simulink model "model_wind_open_loop"  (R2020a)
settings: Solver=ode15s  StartTime=0.0  StopTime=200  MaxStep=1/60  RelTol=1e-2  AbsTol=1e-1  EnableMultiTasking=on
PreLoadFcn:
  | %load_Nordic32_data;
values from neighbouring files (symbols this model uses):
  fn = 50    [load_data_wind_open_loop.m]
  pstep = pstep_(i)    [main_wind_open_loop.m]
  time_event = 45    [load_data_wind_open_loop.m]
  wind_turbines = table(BUS,BSKV,MBASE,POPT,V_WIND,ROT_OPT, ROT_RATED)    [load_data_wind_open_loop.m]
libraries: Nordic32_Lib x2, powerlib x2
settings Model: Creator=Innocent  LastModifiedBy=joakbj
settings SolverCC: AutoScaleAbsTol=off  MaxOrder=2  ZeroCrossAlgorithm=Adaptive
settings DataIOCC: SaveFormat=Array  SaveOutput=off  SaveTime=off  ReturnWorkspaceOutputs=off
settings OptimizationCC: BlockReduction=off  BooleanDataType=off  ExpressionDepthLimit=2147483647  InitFltsAndDblsToZero=on  LifeSpan=inf
settings DebuggingCC: AlgebraicLoopMsg=none  SaveWithParameterizedLinksMsg=none  UnderspecifiedInitializationDetection=Classic  MergeDetectMultiDrivingBlocksExec=none  SignalResolutionControl=TryResolveAllWithWarning  IgnoredZcDiagnostic=none  MultiTaskDSMMsg=warning  MultiTaskCondExecSysMsg=none  FcnCallInpInsideContextMsg=warning  UnconnectedInputMsg=none  UnconnectedOutputMsg=none  UnconnectedLineMsg=none  StateNameClashWarn=warning  StrictBusMsg=ErrorOnBusTreatedAsVector  SFUnexpectedBacktrackingDiag=warning  SFNoUnconditionalDefaultTransitionDiag=warning  SFExecutionAtInitializationDiag=none  ArithmeticOperatorsInVariantConditions=warning
settings HardwareCC: ProdBitPerPointer=32  ProdBitPerSizeT=32  ProdBitPerPtrDiffT=32  ProdLargestAtomicFloat=None  ProdIntDivRoundTo=Undefined  ProdEndianess=Unspecified  ProdWordSize=32  ProdHWDeviceType=32-bit Generic
settings ModelReferenceCC: PropagateSignalLabelsOutOfModel=off
settings SFSimCC: SimUseLocalCustomCode=off  CustomCodeUndefinedFunction=UseInterfaceOnly
settings RTWCC: RTWUseLocalCustomCode=off
settings CodeAppCC: StateflowObjectComments=on
settings GRTTargetCC: TargetFcnLib=ansi_tfl_tmw.mat  TargetLangStandard=C89/C90 (ANSI)  CombineOutputUpdateFcns=off  GRTInterface=on
settings ConfigComp: CovMetricSettings=dw  CovHtmlReporting=on  CovSaveCumulativeToWorkspaceVar=on  CovSaveSingleToWorkspaceVar=on  CovExternalEMLEnable=off
settings SimscapeCC: SimscapeNormalizeSystem=off

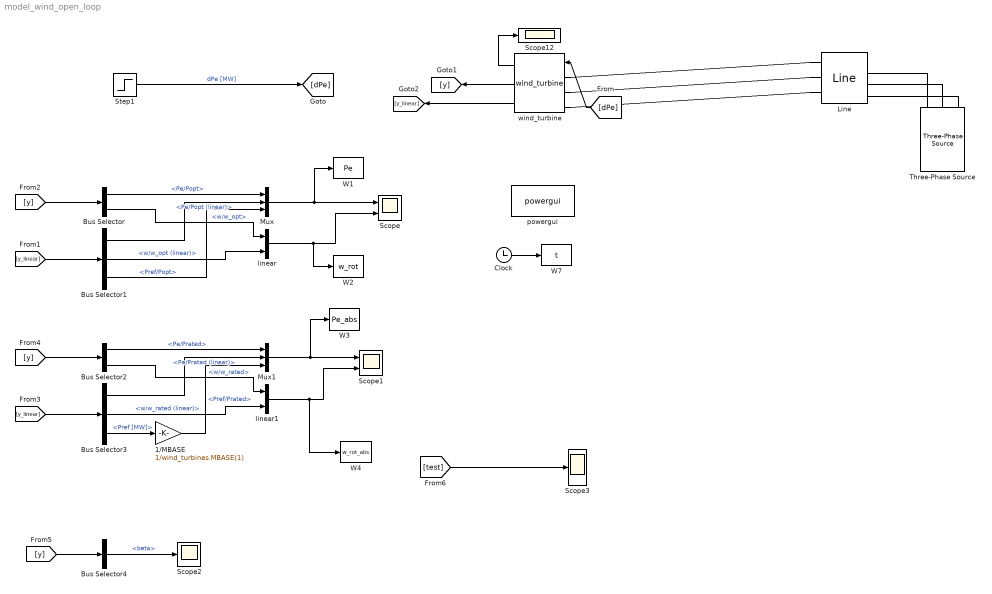
== system model_wind_open_loop ==
  1/MBASE : Gain  Gain=1/wind_turbines.MBASE(1)
  Bus Selector : BusSelector  OutputSignals=Pe/Popt,w/w_opt
  Bus Selector1 : BusSelector  OutputSignals=Pe/Popt (linear),w/w_opt (linear),Pref/Popt
  Bus Selector2 : BusSelector  OutputSignals=Pe/Prated,w/w_rated
  Bus Selector3 : BusSelector  OutputSignals=Pe/Prated (linear),w/w_rated (linear),Pref [MW]
  Bus Selector4 : BusSelector  OutputSignals=beta
  Clock : Clock
  Line : Nordic32_Lib/Line  i=1  data=lines  fn=fn
      link override Distributed Parameters Line: x1=[8.18545231595635e-12 25005.8715597007 25005.8715597007;314.159265358979 314.159265358979 314.159265358979;-0.0355340246434697 0.50191856365132 -1.06887776314358]  x2=[3.74994272134942e-12 25000.0002977636 25000.0002977636;314.159265358979 314.159265358979 314.159265358979;-1.3613516883115 0.501928755329236 -1.06886757146566]  x3=[8.07636853292123e-13 92.3031911494668 92.3031911494664;314.159265358979 314.159265358979 314.159265358979;-2.95655930084788 0.501918563651325 -1.06887776314357]  x4=[8.46150189115196e-13 92.3031860551766 92.303186055177;314.159265358979 314.159265358979 314.159265358979;-2.48934016170634 0.480253191729889 -1.090543135065]  x5=0.000113108313399149
  Mux : Mux  Inputs=3
  Mux1 : Mux  Inputs=3
  Scope : Scope  NumInputPorts=2
  Scope1 : Scope  NumInputPorts=2
  Scope12 : Scope
  Scope2 : Scope
  Scope3 : Scope
  Step1 : Step  Time=time_event  Before=1  After=1-pstep  SampleTime=0
  Three-Phase Source : powerlib/Electrical Sources/Three-Phase Source  InternalConnection=Yg  VoltagePhases=off  Voltage=(25000)*0.999583  PhaseAngle=0.0041233  Voltage_phases=[25e3 25e3 25e3]/sqrt(3)  PhaseAngles_phases=[0 -120 +120]  Frequency=fn  NonIdealSource=on  SpecifyImpedance=off  Resistance=0.8929  Inductance=16.58e-3  ShortCircuitLevel=100e6  BaseVoltage=25e3  XRratio=7  BusType=swing  Pref=10e3  Qref=0  Prefabc=[10e3, 10e3, 10e3]  Qrefabc=[0, 0, 0]  Qmin=-inf  Qmax=inf
  W1 : ToWorkspace  VariableName=Pe  SampleTime=1/60
  W2 : ToWorkspace  VariableName=w_rot  SampleTime=1/60
  W3 : ToWorkspace  VariableName=Pe_abs  SampleTime=1/60
  W4 : ToWorkspace  VariableName=w_rot_abs  SampleTime=1/60
  W7 : ToWorkspace  VariableName=t  SampleTime=1/60
  linear : Mux  Inputs=2
  linear1 : Mux  Inputs=2
  powergui : powerlib/powergui  Priority=2  SimulationMode=Phasor  SampleTime=0  frequency=50  Iterations=100  frequencyindice=50  Pbase=100e6  ErrMax=1e-06  UnitsV=kV  UnitsW=MW  buscounter=3  FunctionMessages=off  echomessages=off  EnableUseOfTLC=off  CurrentSourceSwitches=off  DisableSnubberDevices=off  DisableRonSwitches=off  DisableVfSwitches=off  DisplayEquations=off  AutomaticDiscreteSolvers=off  SolverType=Tustin/Backward Euler (TBE)  Interpol=off  ExternalGateDelay=off  methode=off  Ts=100  x0status=blocks  SPID=off  SwTol=0  HookPort=off  NonlinearTolerance=1e-4  nMaxIteration=100  ContinueOnMaxIteration=off  RestoreLinks=warning  ResistiveCurrentMeasurement=off  Frange=logspace(0,3,50)  Ylog=off  Xlog=off  ShowGrid=off  save=off  variable=ZData  structure=0  ZoomFFT=on  StartTime=0.0  cycles=1  DisplayStyle=1  fundamental=60  FreqAxis=off  MaxFrequency=1000  frequencyindicesteady=1  RmsSteady=1  display=off
  wind_turbine : Nordic32_Lib/wind_turbine  i=1  data=wind_turbines  data_NREL=data_NREL  fn=fn  time_activate_wind=time_activate_wind  Gwind=Gwind  Gwind_speed=Gwind_speed  FCR=tf(1)
      link override Three-Phase Dynamic Load2: ActiveReactivePowers=[0 0]  PositiveSequence=[0.0625147 -0.00061261]
  wires:
  Clock/1 -> W7/1
  wind_turbine/1 -> Scope12/1
  [dPe] -> wind_turbine/1
  wind_turbine/2 -> [y]
  wind_turbine/3 -> [y_linear]
  [y] -> Bus Selector/1
  [y_linear] -> Bus Selector1/1
  Bus Selector/1 -> Mux/1  "<Pe/Popt>"
  Bus Selector1/1 -> Mux/2  "<Pe/Popt (linear)>"
  Bus Selector1/3 -> Mux/3  "<Pref/Popt>"
  Bus Selector/2 -> linear/1  "<w/w_opt>"
  Bus Selector1/2 -> linear/2  "<w/w_opt (linear)>"
  Mux/1 -> W1/1, Scope/1
  linear/1 -> W2/1, Scope/2
  linear1/1 -> W4/1, Scope1/2
  Bus Selector3/2 -> linear1/2  "<w/w_rated (linear)>"
  Bus Selector3/3 -> 1/MBASE/1  "<Pref [MW]>"
  Bus Selector3/1 -> Mux1/2  "<Pe/Prated (linear)>"
  Mux1/1 -> W3/1, Scope1/1
  [y] -> Bus Selector2/1
  Bus Selector2/2 -> linear1/1  "<w/w_rated>"
  [y_linear] -> Bus Selector3/1
  Bus Selector2/1 -> Mux1/1  "<Pe/Prated>"
  1/MBASE/1 -> Mux1/3  "<Pref/Prated>"
  [y] -> Bus Selector4/1
  Bus Selector4/1 -> Scope2/1  "<beta>"
  [test] -> Scope3/1
  Step1/1 -> [dPe]  "dPe [MW]"
  connections:
  Line/LConn1 -- wind_turbine/LConn1
  Line/LConn2 -- wind_turbine/LConn2
  Line/LConn3 -- wind_turbine/LConn3
  Line/RConn1 -- Three-Phase Source/RConn1
  Line/RConn2 -- Three-Phase Source/RConn2
  Line/RConn3 -- Three-Phase Source/RConn3
